simulink model "covert_attack"  (R2021a)
settings: Solver=VariableStepAuto  StartTime=0.0  StopTime=simulation_time  RelTol=1e-3
values from neighbouring files (symbols this model uses):
  a = 50    [compute_fscore_covert.m]    (also in compute_fscore_replay.m; compute_mu_sigma.m = 1/sqrt(det(cov_v_hat)); compute_threshold.m; compute_uio_gain.m = rank([C*E D]))
  b = 150    [compute_fscore_covert.m]    (also in compute_fscore_replay.m; compute_mu_sigma.m = 0.0253302959106; compute_threshold.m; compute_uio_gain.m = rank(E) + rank(D))
  sample_time = 1    [compute_fscore_covert.m]    (also in compute_fscore_replay.m; compute_mu_sigma.m; compute_pcs.m; compute_threshold.m)
  threshold = 0.14    [compute_fscore_covert.m]    (also in compute_fscore_replay.m; compute_mu_sigma.m = 500000000000; compute_pcs.m = 1; compute_threshold.m)
libraries: dspstat3 x1
settings Model: Creator=mehra  LastModifiedBy=mehra

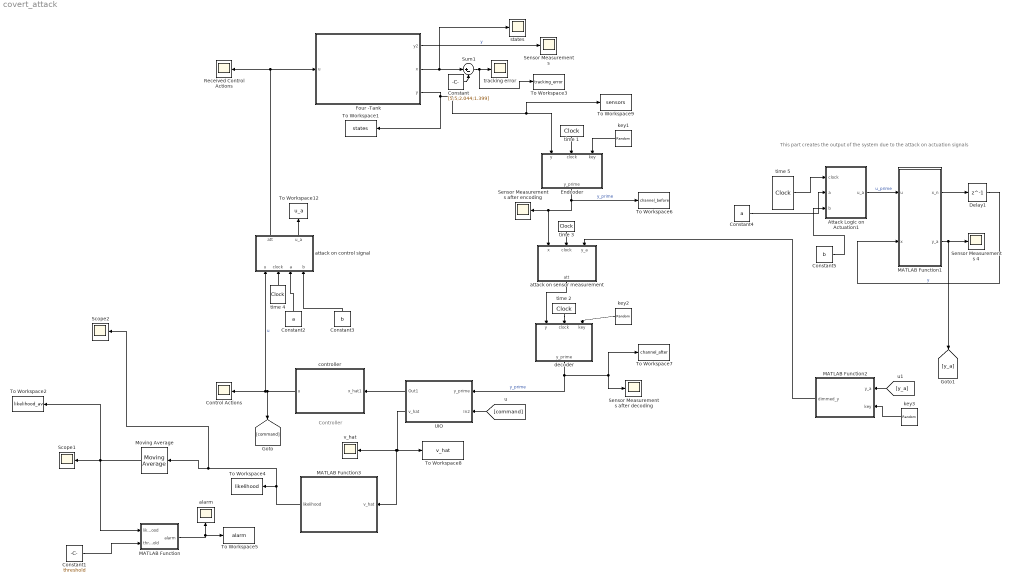
== system covert_attack ==
  note: Controller
  note: This part creates the output of the system due to the attack on actuation signals
  " Control Actions" : Scope
  Attack Logic on Actuation1 : MATLAB Function  TreatAsAtomicUnit=on
  Constant : Constant  Value=[5;5;2.044;1.399]  SampleTime=sample_time
  Constant1 : Constant  Value=threshold  SampleTime=sample_time
  Constant2 : Constant  Value=a  SampleTime=sample_time
  Constant3 : Constant  Value=b  SampleTime=sample_time
  Constant4 : Constant  Value=a  SampleTime=sample_time
  Constant5 : Constant  Value=b  SampleTime=sample_time
  Delay1 : Delay  DelayLength=1  InitialCondition=[0;0;0;0]  SampleTime=sample_time
  "Endcoder " : MATLAB Function  TreatAsAtomicUnit=on
  "Four -Tank " : Subsystem
  MATLAB Function : MATLAB Function  TreatAsAtomicUnit=on
  MATLAB Function1 : MATLAB Function  TreatAsAtomicUnit=on
  MATLAB Function2 : MATLAB Function  TreatAsAtomicUnit=on
  MATLAB Function3 : MATLAB Function  TreatAsAtomicUnit=on
  Moving Average : dspstat3/Moving Average  Method=Sliding window  ForgettingFactorPort=off  SpecifyWindowLength=on  WindowLength=20  ForgettingFactor=0.9  SimulateUsing=Code generation
  Received Control Actions : Scope
  Scope1 : Scope
  Scope2 : Scope
  Sensor Measurements : Scope
  Sensor Measurements 4 : Scope
  Sensor Measurements after decoding : Scope
  Sensor Measurements after encoding : Scope
  Sum1 : Sum  Inputs=|+-
  To Workspace1 : ToWorkspace  VariableName=states  SaveFormat=Timeseries  SampleTime=sample_time
  To Workspace12 : ToWorkspace  VariableName=u_a  SaveFormat=Timeseries  SampleTime=sample_time
  To Workspace2 : ToWorkspace  VariableName=likelihood_av  SaveFormat=Timeseries  SampleTime=sample_time
  To Workspace3 : ToWorkspace  VariableName=tracking_error  SaveFormat=Timeseries  SampleTime=sample_time
  To Workspace4 : ToWorkspace  VariableName=likelihood  SaveFormat=Timeseries  SampleTime=sample_time
  To Workspace5 : ToWorkspace  VariableName=alarm  SaveFormat=Timeseries  SampleTime=sample_time
  To Workspace6 : ToWorkspace  VariableName=channel_before  SaveFormat=Timeseries  SampleTime=sample_time
  To Workspace7 : ToWorkspace  VariableName=channel_after  SaveFormat=Timeseries  SampleTime=sample_time
  To Workspace8 : ToWorkspace  VariableName=v_hat  SaveFormat=Timeseries  SampleTime=sample_time
  To Workspace9 : ToWorkspace  VariableName=sensors  SaveFormat=Timeseries  SampleTime=sample_time
  UIO : Subsystem
  alarm : Scope
  attack on control signal : MATLAB Function  TreatAsAtomicUnit=on
  attack on sensor measurement : MATLAB Function  TreatAsAtomicUnit=on
  controller : MATLAB Function  TreatAsAtomicUnit=on
  decoder : MATLAB Function  TreatAsAtomicUnit=on
  key1 : UniformRandomNumber  Minimum=0  Maximum=4  Seed=20  SampleTime=sample_time
  key2 : UniformRandomNumber  Minimum=0  Maximum=4  Seed=20  SampleTime=sample_time
  key3 : UniformRandomNumber  Minimum=0  Maximum=4  Seed=20  SampleTime=sample_time
  states : Scope
  time {1..5} (5 alike) : DigitalClock  SampleTime=sample_time
  tracking error : Scope
  v_hat : Scope
  wires:
  "Endcoder "/1(y_prime) -> To Workspace6/1, Sensor Measurements after encoding/1, attack on sensor measurement/1(x)  "y_prime"
  UIO/1(Out1) -> controller/1(x_hat1)
  Constant/1 -> Sum1/2
  key2/1 -> decoder/3(key)
  [command] -> UIO/2(In2)
  MATLAB Function3/1(likelihood) -> Scope2/1, Moving Average/1, To Workspace4/1
  attack on control signal/2(u_a) -> To Workspace12/1
  decoder/1(y_prime) -> To Workspace7/1, Sensor Measurements after decoding/1, UIO/1(y_prime)  "y_prime"
  Sum1/1 -> To Workspace3/1, tracking error/1
  key1/1 -> "Endcoder "/3(key)
  "Four -Tank "/2("x ") -> Sum1/1, states/1
  attack on sensor measurement/1(att) -> decoder/1(y)
  Moving Average/1 -> MATLAB Function/1(likelihood), To Workspace2/1, Scope1/1
  time 3/1 -> attack on sensor measurement/2(clock)
  time 1/1 -> "Endcoder "/2(clock)
  "Four -Tank "/3(y) -> To Workspace1/1, To Workspace9/1, "Endcoder "/1(y)
  attack on control signal/1(att) -> Received Control Actions/1, "Four -Tank "/1(u)
  time 4/1 -> attack on control signal/2(clock)
  MATLAB Function/1(alarm) -> alarm/1, To Workspace5/1
  "Four -Tank "/1(y2) -> Sensor Measurements/1  "y"
  Constant1/1 -> MATLAB Function/2(threshold)
  time 2/1 -> decoder/2(clock)
  UIO/2(v_hat) -> To Workspace8/1, MATLAB Function3/1(v_hat), v_hat/1
  controller/1(u) -> " Control Actions"/1, attack on control signal/1(u), [command]  "u"
  [y_a] -> MATLAB Function2/1(y_a)
  key3/1 -> MATLAB Function2/2(key)
  Delay1/1 -> MATLAB Function1/2(x)  "y"
  MATLAB Function2/1(dimmed_y) -> attack on sensor measurement/3(y_a)
  Attack Logic on Actuation1/1(u_a) -> MATLAB Function1/1(u)  "u_prime"
  MATLAB Function1/2(y_a) -> Sensor Measurements 4/1, [y_a]
  time 5/1 -> Attack Logic on Actuation1/1(clock)
  MATLAB Function1/1(x_n) -> Delay1/1
  Constant2/1 -> attack on control signal/3(a)
  Constant3/1 -> attack on control signal/4(b)
  Constant4/1 -> Attack Logic on Actuation1/2(a)
  Constant5/1 -> Attack Logic on Actuation1/3(b)

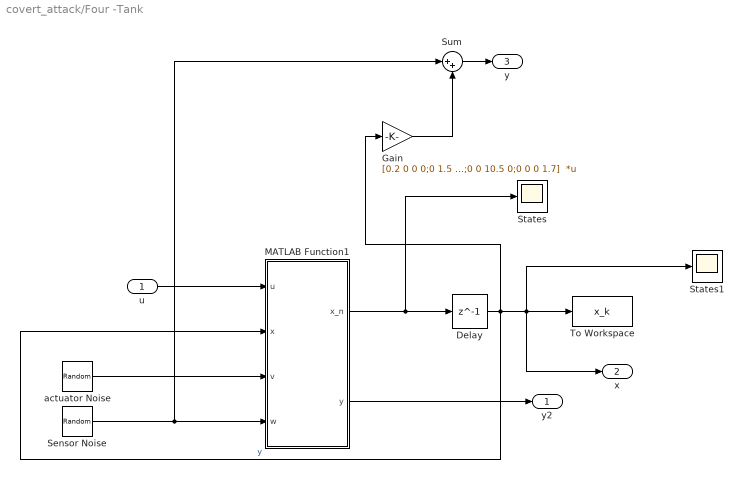
== system covert_attack/Four -Tank  ==
  u : Inport
  Delay : Delay  DelayLength=1  InitialCondition=[5;5;2;1]  SampleTime=sample_time
  Gain : Gain  Gain=[0.2 0 0 0;0 1.5 0 0;0 0 10.5 0;0 0 0 1.7]  Multiplication=Matrix(K*u)
  MATLAB Function1 : MATLAB Function  TreatAsAtomicUnit=on
  Sensor Noise : RandomNumber  Mean=[0 0 0 0]  Variance=[0.00001 0.00001 0.00001 0.00001]  Seed=[randi(100) randi(100) randi(100) randi(100)]  SampleTime=sample_time
  States : Scope
  States1 : Scope
  Sum : Sum  Inputs=|++
  To Workspace : ToWorkspace  VariableName=x_k  SaveFormat=Timeseries  SampleTime=sample_time
  actuator Noise : RandomNumber  Mean=[0 0 0 0]  Variance=[0.00001 0.00001 0.00001 0.00001]  Seed=[randi(100) randi(100) randi(100) randi(100)]  SampleTime=sample_time
  y2 : Outport  VectorParamsAs1DForOutWhenUnconnected=off
  "x " : Outport  Port=2  VectorParamsAs1DForOutWhenUnconnected=off
  y : Outport  Port=3  VectorParamsAs1DForOutWhenUnconnected=off
  wires:
  u/1 -> MATLAB Function1/1(u)
  MATLAB Function1/1(x_n) -> States/1, Delay/1
  MATLAB Function1/2(y) -> y2/1
  Sensor Noise/1 -> Sum/1, MATLAB Function1/4(w)
  actuator Noise/1 -> MATLAB Function1/3(v)
  Delay/1 -> Gain/1, "x "/1, States1/1, To Workspace/1, MATLAB Function1/2(x)  "y"
  Gain/1 -> Sum/2
  Sum/1 -> y/1

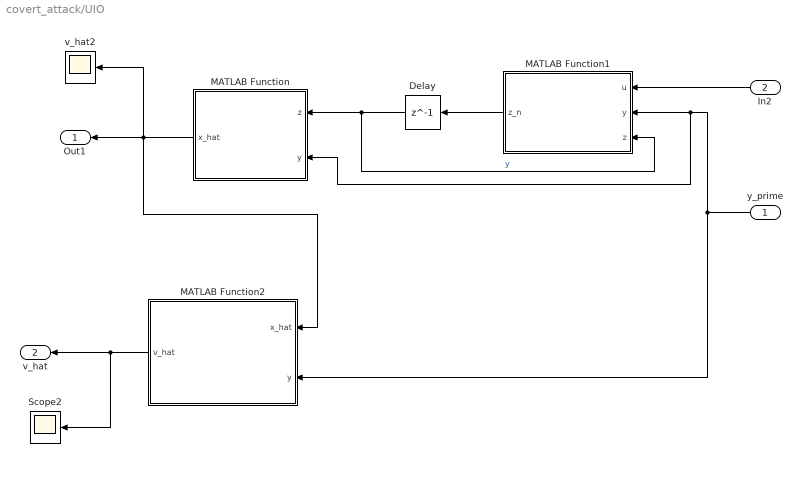
== system covert_attack/UIO ==
  y_prime : Inport
  In2 : Inport  Port=2
  Delay : Delay  DelayLength=1  InitialCondition=[5;5;2;1]  SampleTime=sample_time
  MATLAB Function : MATLAB Function  TreatAsAtomicUnit=on
  MATLAB Function1 : MATLAB Function  TreatAsAtomicUnit=on
  MATLAB Function2 : MATLAB Function  TreatAsAtomicUnit=on
  Scope2 : Scope
  v_hat2 : Scope
  Out1 : Outport  VectorParamsAs1DForOutWhenUnconnected=off
  v_hat : Outport  Port=2  VectorParamsAs1DForOutWhenUnconnected=off
  wires:
  MATLAB Function1/1(z_n) -> Delay/1
  In2/1 -> MATLAB Function1/1(u)
  y_prime/1 -> MATLAB Function/2(y), MATLAB Function1/2(y), MATLAB Function2/2(y)
  Delay/1 -> MATLAB Function1/3(z), MATLAB Function/1(z)  "y"
  MATLAB Function/1(x_hat) -> MATLAB Function2/1(x_hat), v_hat2/1, Out1/1
  MATLAB Function2/1(v_hat) -> Scope2/1, v_hat/1

== matlab function covert_attack/MATLAB Function ==
  data: likelihood input; alarm output; threshold input
function alarm = fcn(likelihood,threshold)

% threshold = 0.8;

if likelihood < threshold
    alarm = 1;
else
    alarm = 0;
end

end

== matlab function covert_attack/Attack Logic on Actuation1 ==
  data: u_a output; clock input; a input; b input
function u_a = fcn(clock,a,b)
% this function should contain the attacker action on the control inputs
if (clock>=0 && clock<100)
    u_a = [0,0]';
elseif clock>=250 && clock<350
    u_a = [clock/a,clock/b]';
else
    u_a = [0,0]';
end

u_a = u_a;

== matlab function covert_attack/MATLAB Function1 ==
  data: x_n output; u input; y_a output; x input
function [x_n, y_a] = fcn(u, x)

A=[0.975 0 0.042 0;0 0.977 0 0.044;0 0 0.958 0;0 0 0 0.956];
B=[0.0515 0.0016;0.0019 0.0447;0 0.0737;0.0850 0];


C=[0.2 0 0 0;0 1.5 0 0;0 0 10.5 0;0 0 0 1.7];
D=[0 0;0 0;0 0;0 0];

x_n = A*x + B*u;
y_a = C*x + D*u;

== matlab function covert_attack/MATLAB Function2 ==
  data: y_a input; dimmed_y output; key input
% function dimmed_y = attack(y_a,key)
% 
% if key<=1
% dimmed_y = [y_a,zeros(4,3)];
% elseif key>1 && key<=2
% dimmed_y = [y_a,zeros(4,3)];
% 
% elseif key>2 && key<=3
% dimmed_y = [y_a,zeros(4,3)];
% 
% else
% dimmed_y = [y_a,zeros(4,3)];
% 
% end
% 
function dimmed_y = attack(y_a,key)

if key<=1
dimmed_y = y_a;
elseif key>1 && key<=2
dimmed_y = y_a;

elseif key>2 && key<=3
dimmed_y = y_a;

else
dimmed_y = y_a;

end

== matlab function covert_attack/Endcoder  ==
  data: y input; y_prime output; clock input; key input
function y_prime = encoder(y,clock,key)
% % this function should contain the attacker action on the sensor
% % measurements


t1 = [-0.3162 0 0 0;
    0.6330 0 0 0;
    -0.5626 0 0 0;
    0.4275 0 0 0];
t2 = [-0.3162 0.7194 0 0;
    0.6330 0.2403 0 0;
    -0.5626 -0.4739 0 0;
    0.4275 -0.4473 0 0];
t3 = [-0.3162 0.7194 0.6169 0;
    0.6330 0.2403 -0.0085 0;
    -0.5626 -0.4739 0.2184 0;
    0.4275 -0.4473 0.7561 0];
t4 = [-0.3162    0.7194    0.6169    0.0442;
    0.6330    0.2403   -0.0085    0.7358;
   -0.5626   -0.4739    0.2184    0.6413;
    0.4275   -0.4473    0.7561   -0.2130];


mean = [0.9988    7.5067   21.4526    2.3840]';
var = [0.0043    0.0265    0.0999    0.0160]';
%
if key<=1
    y_normal = (y - mean) / var;
    y_tilda =  t1' * y_normal;
    y_prime = y_tilda';
%     y_prime  = y_prime;
    
elseif key>1 && key<=2
%     transformation = transforamtion2;
    y_normal = (y - mean) / var;
    y_tilda =  t2' * y_normal;
    y_prime = y_tilda';
%     y_prime  = y_prime;
elseif key>2 && key<=3
    y_normal = (y - mean) / var;
    y_tilda =  t3' * y_normal;
    y_prime = y_tilda';
else
    y_normal = (y - mean) / var;
    y_tilda =  t4' * y_normal;
    y_prime = y_tilda';

% y_prime = y;
end

== matlab function covert_attack/controller ==
  data: x_hat1 input; u output
function u  = Controller(x_hat1)
%two tanks model 
C=[0.2 0 0 0;0 1.5 0 0;0 0 10.5 0;0 0 0 1.7];
A=[0.975 0 0.042 0;0 0.977 0 0.044;0 0 0.958 0;0 0 0 0.956];
B=[0.0515 0.0016;0.0019 0.0447;0 0.0737;0.0850 0];

%controller gain
% K2=[-2.03 -0.0657 -0.0412 -3.2652;-1.0716 -2.3495 -3.7746 -0.0535];

K2=[-0.03 0.0657 -.0412 3.2652;-0.0716 -2.3495 -3.7746 -0.0535];
x_eq=[5;5;2.044;1.399];
u_eq=[0.724;1.165];

u= K2*(x_hat1 - x_eq)+u_eq;

== matlab function covert_attack/UIO/MATLAB Function1 ==
  data: u input; z_n output; y input; z input
function z_n = UIO(u,y,z)

A=[0.975 0 0.042 0;0 0.977 0 0.044;0 0 0.958 0;0 0 0 0.956];
B=[0.0515 0.0016;0.0019 0.0447;0 0.0737;0.0850 0];


C=[0.2 0 0 0;0 1.5 0 0;0 0 10.5 0;0 0 0 1.7];
% D=[0 0;0 0;0 0;0 0];
D = [zeros(4,4) eye(4,4)];

% M = [-0.0488   -0.0294    0.1047   -0.2264;...
%    -0.0488   -0.0294    0.1047   -0.0264;...
%    -0.0488   -0.0294    0.1047   -0.0264;...
%    -0.5488   -0.0294    0.1047   -0.0264];
M = [-0.0488   -0.0294    0.1047   -0.0264;...
   -0.0488   -0.0294    0.1047   -0.0264;...
   -0.0488   -0.0294    0.1047   -0.0264;...
   -0.0488   -0.0294    0.1047   -0.0264];
% OK Gain
% alfa 0.9
L1 = [3.2716    2.5752   -0.0870   -0.7387;...
   -0.1818    1.0351   -0.0989   -0.0544;...
    0.0159    0.0777   -0.0088    0.0117;...
   -0.1437    0.3233   -0.0991    0.5003];

% L = [.49    1.7752   -0.0870   -0.7387;...
%    -0.2818    1.0351   -0.0989   -0.0544;...
%     -0.159    .0777   -0.0088    0.0117;...
%    -0.13437    .3233   -0.0991    0.5003];

% alfa = 0.99 
L2 =[4.0206    1.4720   -0.0910   -0.4066;...
   -0.0780    0.8810   -0.0995   -0.0080;...
    0.0302    0.0565   -0.0089    0.0181;...
   -0.0568    0.1958   -0.0996    0.5387];
% alfa = 0.7;
L3 = [1.4732    3.6086   -0.0835   -1.0706;...
   -0.4313    1.1833   -0.0984   -0.1018;...
   -0.0186    0.0976   -0.0087    0.0053;...
   -0.3520    0.4415   -0.0988    0.4623];

L4 = [4.9226    0.0287   -0.0962    0.0264;...
    0.0476    0.6801   -0.1002    0.0523;...
    0.0476    0.0287   -0.0090    0.0264;...
    0.0476    0.0287   -0.1002    0.5888];

L5 = [4.9710    0.0296   -0.0962    0.0271;...
    0.0543    0.6802   -0.1002    0.0524;...
    0.0485    0.0288   -0.0090    0.0264;...
    0.0532    0.0288   -0.1002    0.5889];

L6 = [4.8050    0.0555   -0.0961    0.0165;...
    0.0315    0.6838   -0.1002    0.0509;...
    0.0453    0.0293   -0.0090    0.0262;...
    0.0338    0.0318   -0.1002    0.5876];

z_n = (eye(4)-M*C)*(A*z + A*M*y+B*u) + L6*(y - C*z - C*M*y);

x_hat = z + M*y;

== matlab function covert_attack/UIO/MATLAB Function ==
  data: z input; x_hat output; y input
function x_hat = estimator(z,y)

% M = [-0.0488   -0.0294    0.1047   -0.0264;...
%    -0.0488   -0.0294    0.1047   -0.0264;...
%    -0.0488   -0.0294    0.1047   -0.0264;...
%    -0.0488   -0.0294    0.1047   -0.0264];

M = [-0.0488   -0.0294    0.1047   -0.0264;...
   -0.0488   -0.0294    0.1047   -0.0264;...
   -0.0488   -0.0294    0.1047   -0.0264;...
   -0.0488   -0.0294    0.1047   -0.0264];

x_hat = z + M*y;

== matlab function covert_attack/Four -Tank /MATLAB Function1 ==
  data: x_n output; u input; y output; x input; v input; w input
function [x_n, y] = fcn(u, x, v, w)


A=[0.975 0 0.042 0;0 0.977 0 0.044;0 0 0.958 0;0 0 0 0.956];
B=[0.0515 0.0016;0.0019 0.0447;0 0.0737;0.0850 0];
C=[0.2 0 0 0;0 1.5 0 0;0 0 10.5 0;0 0 0 1.7];
D=[0 0;0 0;0 0;0 0];


x_n = A*x + B*u + v;
y = C*x + D*u + w;

== matlab function covert_attack/UIO/MATLAB Function2 ==
  data: x_hat input; v_hat output; y input
function v_hat = unknown_estimator(x_hat,y)

C = [0.2 0 0 0;0 1.5 0 0;0 0 10.5 0;0 0 0 1.7];
% D = [0.5;0.5;0.5;0.5];
D = [zeros(4,4) eye(4,4)];
q = pinv(D)*y - pinv(D)*C*x_hat;
v_hat = q(5:8);

== matlab function covert_attack/MATLAB Function3 ==
  data: v_hat input; likelihood output
function likelihood  = Anomaly_Detector(v_hat)


cov = 1.0e-03 * [0.0017    0.0142    0.0085    0.0144;
    0.0142    0.1369    0.0745    0.1148;
    0.0085    0.0745    0.0428    0.0699;
    0.0144    0.1148    0.0699    0.1210];

mean = 1.0e-03 * [0.2571   -0.4191    0.1378    0.5351]';

a = 1.3256e+15;
b = 0.0253;

% likelihood = a * b *exp(-0.5*(v_hat-mean)' * inv(cov) * (v_hat-mean));
likelihood = exp(-0.5*(v_hat-mean)' * inv(cov) * (v_hat-mean));


end

== matlab function covert_attack/decoder ==
  data: y input; y_prime output; clock input; key input
function y_prime  = decoder(y,clock,key)
% % this function should contain the attacker action on the sensor

t1 = [-0.3162 0 0 0;
    0.6330 0 0 0;
    -0.5626 0 0 0;
    0.4275 0 0 0];
t2 = [-0.3162 0.7194 0 0;
    0.6330 0.2403 0 0;
    -0.5626 -0.4739 0 0;
    0.4275 -0.4473 0 0];
t3 = [-0.3162 0.7194 0.6169 0;
    0.6330 0.2403 -0.0085 0;
    -0.5626 -0.4739 0.2184 0;
    0.4275 -0.4473 0.7561 0];
t4 = [-0.3162    0.7194    0.6169    0.0442;
    0.6330    0.2403   -0.0085    0.7358;
   -0.5626   -0.4739    0.2184    0.6413;
    0.4275   -0.4473    0.7561   -0.2130];


mean = [0.9988    7.5067   21.4526    2.3840]';
var = [0.0043    0.0265    0.0999    0.0160]';


if key<=1
%     transformation = transformation1;
    y_recons = y * (t1');
    y_hat = (y_recons * var) + mean;
    y_prime = y_hat;
elseif key>1 && key<=2

%     transformation = transformation2;
    y_recons = y * (t2');
    y_hat = (y_recons * var) + mean;
    y_prime = y_hat;
elseif key>2 && key<=3
    y_recons = y * (t3');
    y_hat = (y_recons * var) + mean;
    y_prime = y_hat;
    
else
    y_recons = y * (t4');
    y_hat = (y_recons * var) + mean;
    y_prime = y_hat;
%     
% y_prime = y;
end

== matlab function covert_attack/attack on sensor measurement ==
  data: x input; att output; clock input; y_a input
function att = attack(x,clock,y_a)
if clock<250
    att = x;
elseif clock>=250&& clock<=350
   att = x - [y_a, y_a, y_a, y_a];
%    att = x;
else
    att = x;

end

== matlab function covert_attack/attack on control signal ==
  data: u input; att output; clock input; u_a output; a input; b input
function [att,u_a] = attack(u,clock,a,b)
if clock<250
    att = u;
    u_a = 0;
elseif clock>=250&& clock<=350
    att = u + [clock/a; clock/b];
    u_a = 1;
%     att = u;
else
    att = u;
    u_a = 0;
end
